simulink model "train"  (R2017a)
settings: Solver=ode45  StartTime=0.0  StopTime=1000  RelTol=1e-3
values from neighbouring files (symbols this model uses):
  g = 9.8    [train_script.m]
  k = 1    [train_script.m]
  M1 = 1    [train_script.m]
  M2 = 0.5    [train_script.m]
  mu = 0.02    [train_script.m]
settings Model: Creator=sansh  LastModifiedBy=sansh

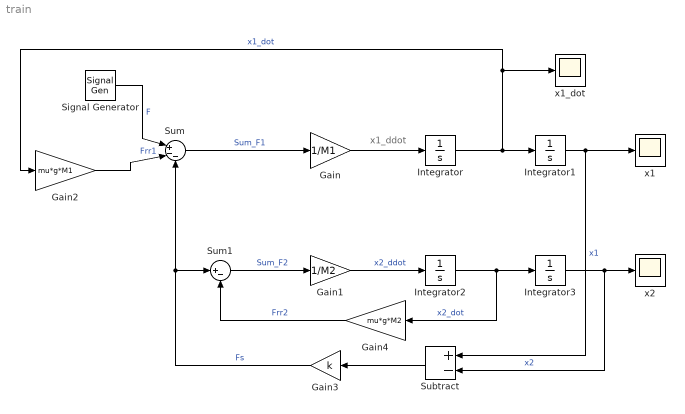
== system train ==
  note: x1_ddot
  Gain : Gain  Gain=1/M1
  Gain1 : Gain  Gain=1/M2
  Gain2 : Gain  Gain=mu*g*M1
  Gain3 : Gain  Gain=k
  Gain4 : Gain  Gain=mu*g*M2
  Integrator{,1..3} (4 alike) : Integrator
  Signal Generator : SignalGenerator  WaveForm=square  Amplitude=-1  Frequency=0.001
  Subtract : Sum  Inputs=+-
  Sum : Sum  Inputs=|+--
  Sum1 : Sum  Inputs=|+-
  x1 : Scope
  x1_dot : Scope
  x2 : Scope
  wires:
  Sum/1 -> Gain/1  "Sum_F1"
  Sum1/1 -> Gain1/1  "Sum_F2"
  Gain/1 -> Integrator/1
  Integrator/1 -> x1_dot/1, Gain2/1, Integrator1/1  "x1_dot"
  Gain1/1 -> Integrator2/1  "x2_ddot"
  Integrator2/1 -> Gain4/1, Integrator3/1  "x2_dot"
  Integrator1/1 -> Subtract/1, x1/1  "x1"
  Integrator3/1 -> Subtract/2, x2/1  "x2"
  Signal Generator/1 -> Sum/1  "F"
  Gain2/1 -> Sum/2  "Frr1"
  Subtract/1 -> Gain3/1
  Gain3/1 -> Sum1/1, Sum/3  "Fs"
  Gain4/1 -> Sum1/2  "Frr2"
